simulink model "platform_dp_2021b"  (R2021b)
settings: Solver=ode4  StartTime=0.0  StopTime=500  FixedStep=0.05  RelTol=1e-3
values from neighbouring files (symbols this model uses):
  Kd = 3*alpha_r-beta_r    [kod.m]
  Kd_pos_surge = 0.1    [kod.m]
  Kd_pos_sway = 0.1    [kod.m]
  Ki = alpha_r    [kod.m]
  Ki_vel_surge = alpha_u    [kod.m]
  Ki_vel_sway = alpha_v    [kod.m]
  Kp = 3*alpha_r    [kod.m]
  Kp_pos_surge = 0.05    [kod.m]
  Kp_pos_sway = 0.05    [kod.m]
  Kp_vel_surge = 2*alpha_u    [kod.m]
  Kp_vel_sway = 2*alpha_v    [kod.m]
  limit_max = 2.2    [kod.m]
  limit_min = -limit_max    (= -2.2)    [kod.m]
  pocetni_surge = 1    [kod.m]
  pocetni_sway = 1    [kod.m]
undefined symbols (not defined in the file or in its folder): t200_force, t200_rps
libraries: LABUST_library x7
settings Model: Creator=thor  LastModifiedBy=Filip
settings DataIOCC: SaveFormat=Array  SignalLogging=off  DSMLogging=off  ReturnWorkspaceOutputs=off

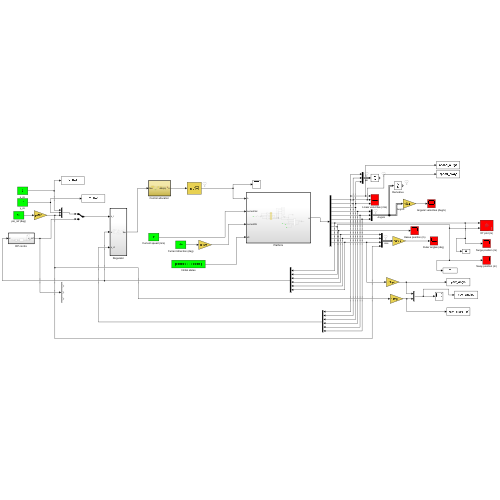
[thumbnail: Simulink's stored preview of the top-level diagram]
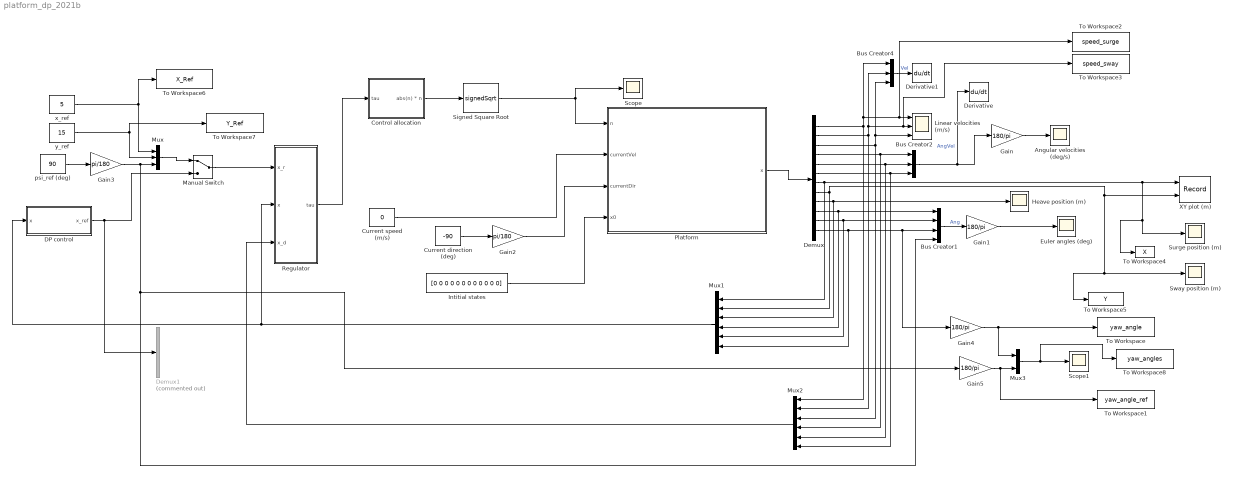
== system platform_dp_2021b ==
  Angular velocities (deg/s) : Scope
  Bus Creator1 : BusCreator  Inputs=4
  Bus Creator2 : BusCreator  Inputs=3
  Bus Creator4 : BusCreator  Inputs=3
  Control allocation : Subsystem  TreatAsAtomicUnit=on
  Current direction (deg) : Constant  Value=-90
  Current speed (m/s) : Constant  Value=0
  DP control : Subsystem  TreatAsAtomicUnit=on
      settings: MinAlgLoopOccurrences=on
  Demux : Demux  Outputs=12
  Demux1 : Demux  Commented=on  Outputs=3
  Derivative : Derivative
  Derivative1 : Derivative
  Euler angles (deg) : Scope
  Gain{,1,4..5} (4 alike) : Gain  Gain=180/pi
  Gain2 : Gain  Gain=pi/180
  Gain3 : Gain  Gain=pi/180
  Heave position (m) : Scope
  Intitial states : Constant  Value=[0 0 0 0 0 0 0 0 0 0 0 0]
  Linear velocities (m/s) : Scope  NumInputPorts=3
  Manual Switch : ManualSwitch
  Mux : Mux  Inputs=3
  Mux1 : Mux  Inputs=6
  Mux2 : Mux  Inputs=6
  Mux3 : Mux  Inputs=2
  Platform : Subsystem  TreatAsAtomicUnit=on
      settings: MinAlgLoopOccurrences=on
  Regulator : Subsystem  TreatAsAtomicUnit=on
  Scope : Scope
  Scope1 : Scope
  Signed Square Root : Sqrt  Operator=signedSqrt  SaturateOnIntegerOverflow=on
  Surge position (m) : Scope
  Sway position (m) : Scope
  To Workspace : ToWorkspace  VariableName=yaw_angle  SaveFormat=Timeseries  SampleTime=-1
  To Workspace1 : ToWorkspace  VariableName=yaw_angle_ref  SaveFormat=Timeseries  SampleTime=-1
  To Workspace2 : ToWorkspace  VariableName=speed_surge  SaveFormat=Timeseries  SampleTime=-1
  To Workspace3 : ToWorkspace  VariableName=speed_sway  SaveFormat=Timeseries  SampleTime=-1
  To Workspace4 : ToWorkspace  VariableName=X  SaveFormat=Timeseries  SampleTime=-1
  To Workspace5 : ToWorkspace  VariableName=Y  SaveFormat=Timeseries  SampleTime=-1
  To Workspace6 : ToWorkspace  VariableName=X_Ref  SaveFormat=Timeseries  SampleTime=-1
  To Workspace7 : ToWorkspace  VariableName=Y_Ref  SaveFormat=Timeseries  SampleTime=-1
  To Workspace8 : ToWorkspace  VariableName=yaw_angles  SaveFormat=Timeseries  SampleTime=-1
  XY plot (m) : Record  FileSettingsInternal="{\"entries\":[{\"content\":{\"excelSettings\":{\"content\":{},\"type\":\"Streamout.ExcelSettings\"}},\"type\":\"Streamout.FileSettingStorage\",\"uuid\":\"f6c939ad-3c6c-47f6-b630-397268ba4e02\"}],\"packageUris\":[\"http://schema.mathworks.com/mf0/streamout_blocks/R2020a\"],\"version\":\"1.0\"}"  Layout=[1 1]  SignalsInternal="{\"entries\":[{\"content\":{\"signals\":[{\"content\":{\"blockPath\":[\"platform_dp_2021b/XY plot (m)\"],\"channel\":[],\"dimensions\":[1],\"domain\":\"platform_dp_2021b/XY plot (m)\",\"lineColor\":\"#a2142f\",\"plots\":[1],\"port\":1,\"sid\":[],\"signalID\":26,\"signalName\":\"Demux:7\"},\"type\":\"RecordBlkView.Signal\",\"uuid\":\"c9e5ced9-c3c6-4cfe-b485-63496ada43a6\"},{\"content\":{\"blockPath\":[\"platform_dp_2021b/XY plot (m)\"],\"channel\":[],\"dimensions\":[1],\"domain\":\"platform_dp_2021b/XY plot (m)\",\"lineColor\":\"#139fff\",\"plots\":[1],\"port\":2,\"sid\":[],\"signalID\":29,\"signalName\":\"Demux:8\"},\"type\":\"RecordBlkView.Signal\",\"uuid\":\"c26e96c1-7e93-4fdd-b2af-f7d2bbcdf98a\"}]},\"type\":\"RecordBlkView.InputSignals\",\"uuid\":\"881e7a22-5157-46d7-a09a-0495ef89bb52\"}],\"packageUris\":[\"http://schema.mathworks.com/mf0/streamout_blocks/R2020a\"],\"version\":\"1.0\"}"  VisualizationBindings="{\"xyplotplugin\":{\"info\":[{\"series\":[{\"bindingParametersList\":[{\"parameter\":\"X-Axis\",\"signalID\":26,\"signalName\":\"Demux:7\"},{\"parameter\":\"Y-Axis\",\"signalID\":29,\"signalName\":\"Demux:8\"}],\"seriesID\":55077}],\"subplotID\":1}]}}"  CompatibilityTag=XY  st=-1
  psi_ref (deg) : Constant  Value=90
  x_ref : Constant  Value=5
  y_ref : Constant  Value=15
  wires:
  Demux/1 -> Bus Creator4/1, To Workspace2/1, Linear velocities (m/s)/1, Mux2/1
  Demux/2 -> To Workspace3/1, Linear velocities (m/s)/2, Bus Creator4/2, Mux2/2
  Demux/3 -> Linear velocities (m/s)/3, Bus Creator4/3, Mux2/3
  Demux/4 -> Mux2/4, Bus Creator2/1
  Demux/5 -> Mux2/5, Bus Creator2/2
  Bus Creator2/1 -> Derivative/1, Gain/1  "AngVel"
  Current speed (m/s)/1 -> Platform/2(currentVel)
  Current direction (deg)/1 -> Gain2/1
  Intitial states/1 -> Platform/4(x0)
  Gain/1 -> Angular velocities (deg/s)/1
  Gain1/1 -> Euler angles (deg)/1
  Gain2/1 -> Platform/3(currentDir)
  Demux/6 -> Mux2/6, Bus Creator2/3
  Gain3/1 -> Mux/3, Gain5/1, Bus Creator1/4
  Bus Creator1/1 -> Gain1/1  "Ang"
  Control allocation/1(abs(n) * n) -> Signed Square Root/1
  Bus Creator4/1 -> Derivative1/1  "Vel"
  y_ref/1 -> To Workspace7/1, Mux/2
  Mux2/1 -> Regulator/3(x_d)
  Platform/1(x) -> Demux/1
  Signed Square Root/1 -> Platform/1(n), Scope/1
  Regulator/1(tau) -> Control allocation/1(tau)
  Mux/1 -> Manual Switch/1
  Manual Switch/1 -> Regulator/1(x_r)
  DP control/1(x_ref) -> Demux1/1, Manual Switch/2
  Mux1/1 -> DP control/1(x), Regulator/2(x)
  Demux/7 -> Mux1/1, Surge position (m)/1, To Workspace4/1, XY plot (m)/1
  Demux/8 -> To Workspace5/1, Sway position (m)/1, XY plot (m)/2, Mux1/2
  Demux/9 -> Mux1/3, Heave position (m)/1
  Demux/10 -> Mux1/4, Bus Creator1/1
  Demux/11 -> Mux1/5, Bus Creator1/2
  Demux/12 -> Mux1/6, Gain4/1, Bus Creator1/3
  psi_ref (deg)/1 -> Gain3/1
  Gain4/1 -> Mux3/1, To Workspace/1
  Mux3/1 -> To Workspace8/1, Scope1/1
  Gain5/1 -> To Workspace1/1, Mux3/2
  x_ref/1 -> To Workspace6/1, Mux/1

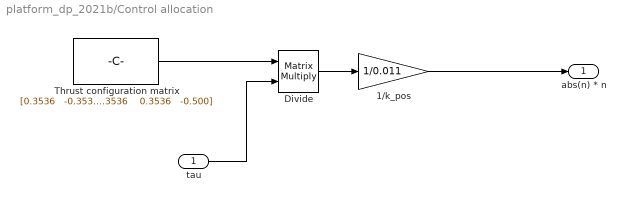
== system platform_dp_2021b/Control allocation ==
  tau : Inport
  1/k_pos : Gain  Gain=1/0.011
  Divide : Product  Inputs=**  Multiplication=Matrix(*)
  Thrust configuration matrix : Constant  Value=|
      | [0.3536   -0.3536   -0.500; 0.3536    0.3536    0.500; -0.3536   -0.3536    0.500
      | ; -0.3536    0.3536   -0.500]
  abs(n) * n : Outport
  wires:
  tau/1 -> Divide/2
  Divide/1 -> 1/k_pos/1
  1/k_pos/1 -> abs(n) * n/1
  Thrust configuration matrix/1 -> Divide/1

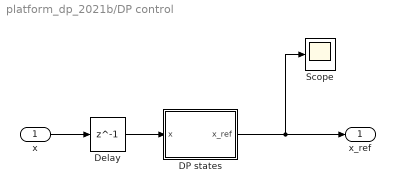
== system platform_dp_2021b/DP control ==
  x : Inport
  DP states : MATLAB Function  TreatAsAtomicUnit=on
  Delay : Delay  DelayLength=1
  Scope : Scope
  x_ref : Outport
  wires:
  x/1 -> Delay/1
  DP states/1(x_ref) -> Scope/1, x_ref/1
  Delay/1 -> DP states/1(x)

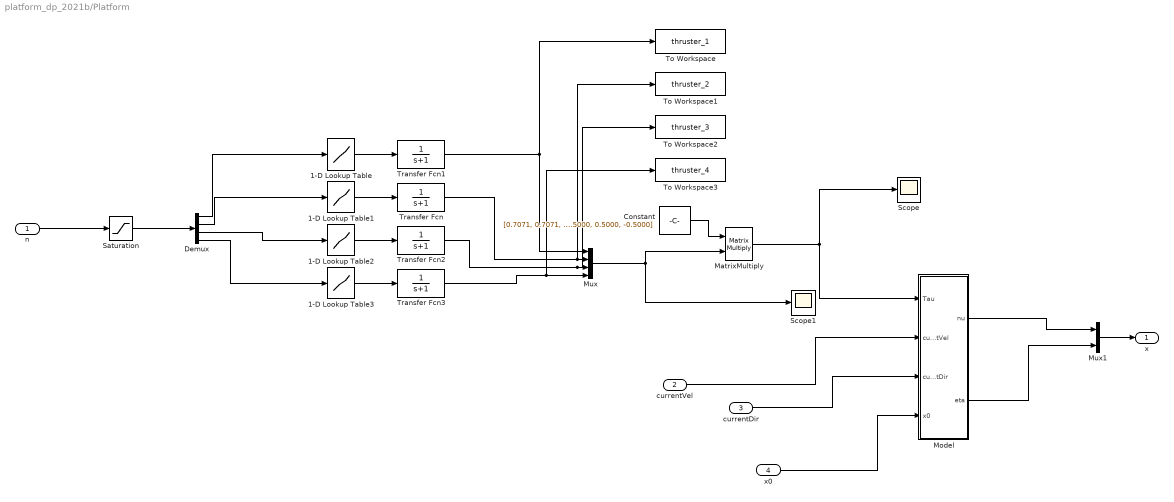
== system platform_dp_2021b/Platform ==
  n : Inport
  currentVel : Inport  Port=2
  currentDir : Inport  Port=3
  x0 : Inport  Port=4
  1-D Lookup Table{,1..3} (4 alike) : Lookup_n-D  NumberOfTableDimensions=1  BreakpointsForDimension1=t200_rps  Table=t200_force  InternalRulePriority=Speed  RndMeth=Simplest  InputSameDT=on
  Constant : Constant  Value="[0.7071, 0.7071, -0.7071, -0.7071; -0.7071,  0.7071, -0.7071,  0.7071; -0.5000, 0.5000, 0.5000, -0.5000]"
  Demux : Demux
  MatrixMultiply : Product  Multiplication=Matrix(*)
  Model : Subsystem
  Mux : Mux
  Mux1 : Mux  Inputs=2
  Saturation : Saturate  UpperLimit=60  LowerLimit=-60
  Scope : Scope
  Scope1 : Scope
  To Workspace : ToWorkspace  VariableName=thruster_1  SaveFormat=Timeseries  SampleTime=-1
  To Workspace1 : ToWorkspace  VariableName=thruster_2  SaveFormat=Timeseries  SampleTime=-1
  To Workspace2 : ToWorkspace  VariableName=thruster_3  SaveFormat=Timeseries  SampleTime=-1
  To Workspace3 : ToWorkspace  VariableName=thruster_4  SaveFormat=Timeseries  SampleTime=-1
  Transfer Fcn{,1..3} (4 alike) : TransferFcn  Denominator=[1 1]
  x : Outport
  wires:
  Transfer Fcn1/1 -> To Workspace/1, Mux/1
  Transfer Fcn/1 -> To Workspace1/1, Mux/2
  Demux/1 -> 1-D Lookup Table/1
  currentVel/1 -> Model/2(currentVel)
  n/1 -> Saturation/1
  Model/1(nu) -> Mux1/1
  Transfer Fcn2/1 -> To Workspace2/1, Mux/3
  Transfer Fcn3/1 -> To Workspace3/1, Mux/4
  Constant/1 -> MatrixMultiply/1
  Mux/1 -> MatrixMultiply/2, Scope1/1
  Model/2(eta) -> Mux1/2
  Mux1/1 -> x/1
  currentDir/1 -> Model/3(currentDir)
  x0/1 -> Model/4(x0)
  MatrixMultiply/1 -> Scope/1, Model/1(Tau)
  Saturation/1 -> Demux/1
  1-D Lookup Table/1 -> Transfer Fcn1/1
  1-D Lookup Table1/1 -> Transfer Fcn/1
  Demux/2 -> 1-D Lookup Table1/1
  Demux/3 -> 1-D Lookup Table2/1
  Demux/4 -> 1-D Lookup Table3/1
  1-D Lookup Table2/1 -> Transfer Fcn2/1
  1-D Lookup Table3/1 -> Transfer Fcn3/1

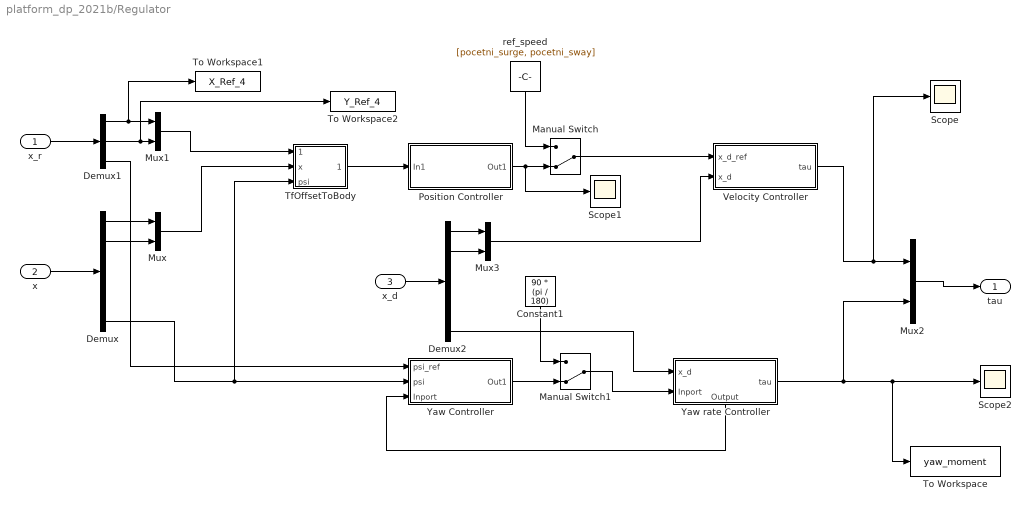
== system platform_dp_2021b/Regulator ==
  x_r : Inport
  x : Inport  Port=2
  x_d : Inport  Port=3
  Constant1 : Constant  Value=90 * (pi / 180)
  Demux : Demux  Outputs=6
  Demux1 : Demux  Outputs=3
  Demux2 : Demux  Outputs=6
  Manual Switch : ManualSwitch  CurrentSetting=0
  Manual Switch1 : ManualSwitch  CurrentSetting=0
  Mux{,1..3} (4 alike) : Mux  Inputs=2
  Position Controller : Subsystem
  Scope : Scope
  Scope1 : Scope
  Scope2 : Scope
  TfOffsetToBody : Subsystem
  To Workspace : ToWorkspace  VariableName=yaw_moment  SaveFormat=Timeseries  SampleTime=-1
  To Workspace1 : ToWorkspace  VariableName=X_Ref_4  SaveFormat=Timeseries  SampleTime=-1
  To Workspace2 : ToWorkspace  VariableName=Y_Ref_4  SaveFormat=Timeseries  SampleTime=-1
  Velocity Controller : Subsystem
  Yaw Controller : Subsystem
  Yaw rate Controller : Subsystem
      settings: PortSchema="{\"entries\":[{\"content\":{\"sides\":[{\"content\":{\"connectorIds\":[\"In1\",\"In2\"]},\"type\":\"ConnectorPlacement.EquallySpacedRectSide\",\"uuid\":\"a08ad913-1b5f-4804-936b-9df89e924933\"},{\"content\":{\"connectorIds\":[\"Out1\"],\"side\":\"RIGHT\"},\"type\":\"ConnectorPlacement.EquallySpacedRectSide\",\"uuid\":\"6b85309d-1e4c-4a26-aaae-a68e51ddcc12\"},{\"content\":{\"connectorIds\":[],\"side\":\"TOP\"},\"type\":\"ConnectorPlacement.EquallySpacedRectSide\",\"uuid\":\"52d97ae7-08e9-4468-b813-b96210971f31\"},{\"content\":{\"connectorIds\":[\"Out2\"],\"side\":\"BOTTOM\"},\"type\":\"ConnectorPlacement.EquallySpacedRectSide\",\"uuid\":\"7dbeefe3-e37d-4eaa-a945-6bd75ab68883\"}]},\"type\":\"ConnectorPlacement.EquallySpacedConnector\",\"uuid\":\"70f5cb1b-651c-4d9e-bb57-ada13c3f9021\"}],\"packageUris\":[\"http://schema.mathworks.com/mf0/Connector/R2020b\"],\"version\":\"1.0\"}"
  ref_speed : Constant  Value=[pocetni_surge, pocetni_sway]
  tau : Outport
  wires:
  TfOffsetToBody/1(Out1) -> Position Controller/1(In1)
  Manual Switch/1 -> Velocity Controller/1(x_d_ref)
  Velocity Controller/1(tau) -> Scope/1, Mux2/1
  Mux3/1 -> Velocity Controller/2(x_d)
  x/1 -> Demux/1
  Demux/1 -> Mux/1
  Demux/2 -> Mux/2
  Mux/1 -> TfOffsetToBody/2(x)
  x_r/1 -> Demux1/1
  Demux1/2 -> To Workspace2/1, Mux1/2
  Mux1/1 -> TfOffsetToBody/1(x_ref)
  Yaw rate Controller/1(tau) -> To Workspace/1, Scope2/1, Mux2/2
  Demux1/3 -> Yaw Controller/1(psi_ref)
  Mux2/1 -> tau/1
  Demux/6 -> TfOffsetToBody/3(psi), Yaw Controller/2(psi)
  Demux2/1 -> Mux3/1
  x_d/1 -> Demux2/1
  Demux2/2 -> Mux3/2
  Demux1/1 -> To Workspace1/1, Mux1/1
  Position Controller/1(Out1) -> Scope1/1, Manual Switch/2
  ref_speed/1 -> Manual Switch/1
  Constant1/1 -> Manual Switch1/1
  Yaw rate Controller/2(Output) -> Yaw Controller/3(Inport)
  Demux2/6 -> Yaw rate Controller/1(x_d)
  Yaw Controller/1(Out1) -> Manual Switch1/2
  Manual Switch1/1 -> Yaw rate Controller/2(Inport)

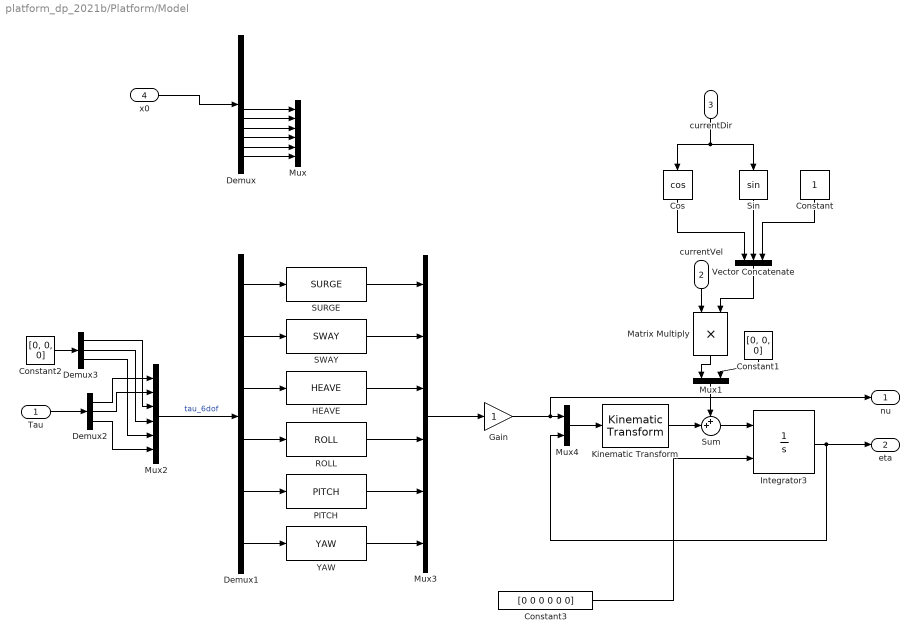
== system platform_dp_2021b/Platform/Model ==
  Tau : Inport
  currentVel : Inport  Port=2
  currentDir : Inport  Port=3
  x0 : Inport  Port=4
  " HEAVE" : LABUST_library/Vehicles/Uncoupled 6DOF/ HEAVE  SystemSampleTime=-1  VariantActivationTime=update diagram  Latency=0  AutoFrameSizeCalculation=off
  " PITCH" : LABUST_library/Vehicles/Uncoupled 6DOF/ PITCH  SystemSampleTime=-1  VariantActivationTime=update diagram  Latency=0  AutoFrameSizeCalculation=off
  " ROLL" : LABUST_library/Vehicles/Uncoupled 6DOF/ ROLL  SystemSampleTime=-1  VariantActivationTime=update diagram  Latency=0  AutoFrameSizeCalculation=off
  " SURGE" : LABUST_library/Vehicles/Uncoupled 6DOF/ SURGE  SystemSampleTime=-1  VariantActivationTime=update diagram  Latency=0  AutoFrameSizeCalculation=off
  " SWAY" : LABUST_library/Vehicles/Uncoupled 6DOF/ SWAY  SystemSampleTime=-1  VariantActivationTime=update diagram  Latency=0  AutoFrameSizeCalculation=off
  " YAW" : LABUST_library/Vehicles/Uncoupled 6DOF/ YAW  SystemSampleTime=-1  VariantActivationTime=update diagram  Latency=0  AutoFrameSizeCalculation=off
  Constant : Constant
  Constant1 : Constant  Value=[0, 0, 0]
  Constant2 : Constant  Value=[0, 0, 0]
  Constant3 : Constant  Value=[0 0 0 0 0 0]
  Cos : Trigonometry  Operator=cos
  Demux : Demux  Outputs=12
  Demux1 : Demux  Outputs=6
  Demux2 : Demux  Outputs=3
  Demux3 : Demux  Outputs=3
  Gain : Gain
  Integrator3 : Integrator  InitialConditionSource=external
  Kinematic Transform : LABUST_library/Vehicles/Uncoupled 6DOF/Kinematic Transform  SystemSampleTime=-1  VariantActivationTime=update diagram  Latency=0  AutoFrameSizeCalculation=off
  Matrix Multiply : Product
  Mux : Mux  Inputs=6
  Mux1 : Mux  Inputs=2
  Mux2 : Mux  Inputs=6
  Mux3 : Mux  Inputs=6
  Mux4 : Mux  Inputs=2
  Sin : Trigonometry
  Sum : Sum  Inputs=++|
  Vector Concatenate : Concatenate  NumInputs=3
  nu : Outport
  eta : Outport  Port=2
  wires:
  Demux1/1 -> " SURGE"/1
  " PITCH"/1 -> Mux3/5
  Mux3/1 -> Gain/1
  " SURGE"/1 -> Mux3/1
  Sum/1 -> Integrator3/1
  Demux1/5 -> " PITCH"/1
  Integrator3/1 -> Mux4/2, eta/1
  Demux1/3 -> " HEAVE"/1
  " HEAVE"/1 -> Mux3/3
  Mux4/1 -> Kinematic Transform/1
  Demux1/4 -> " ROLL"/1
  Demux1/2 -> " SWAY"/1
  " YAW"/1 -> Mux3/6
  Kinematic Transform/1 -> Sum/2
  Gain/1 -> Mux4/1, nu/1
  Demux1/6 -> " YAW"/1
  " SWAY"/1 -> Mux3/2
  " ROLL"/1 -> Mux3/4
  currentVel/1 -> Matrix Multiply/1
  x0/1 -> Demux/1
  currentDir/1 -> Cos/1, Sin/1
  Cos/1 -> Vector Concatenate/1
  Sin/1 -> Vector Concatenate/2
  Constant/1 -> Vector Concatenate/3
  Vector Concatenate/1 -> Matrix Multiply/2
  Demux/7 -> Mux/1
  Demux/8 -> Mux/2
  Demux/9 -> Mux/3
  Demux/10 -> Mux/4
  Demux/11 -> Mux/5
  Demux/12 -> Mux/6
  Matrix Multiply/1 -> Mux1/1
  Constant1/1 -> Mux1/2
  Mux1/1 -> Sum/1
  Tau/1 -> Demux2/1
  Demux2/1 -> Mux2/1
  Demux2/2 -> Mux2/2
  Demux2/3 -> Mux2/6
  Constant2/1 -> Demux3/1
  Demux3/1 -> Mux2/3
  Demux3/2 -> Mux2/4
  Demux3/3 -> Mux2/5
  Mux2/1 -> Demux1/1  "tau_6dof"
  Constant3/1 -> Integrator3/2

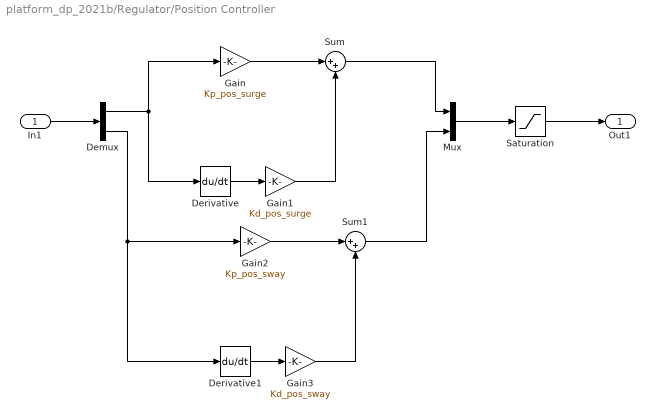
== system platform_dp_2021b/Regulator/Position Controller ==
  In1 : Inport
  Demux : Demux  Outputs=2
  Derivative : Derivative
  Derivative1 : Derivative
  Gain : Gain  Gain=Kp_pos_surge
  Gain1 : Gain  Gain=Kd_pos_surge
  Gain2 : Gain  Gain=Kp_pos_sway
  Gain3 : Gain  Gain=Kd_pos_sway
  Mux : Mux  Inputs=2
  Saturation : Saturate  UpperLimit=2.2  LowerLimit=-2.2
  Sum : Sum  Inputs=|++
  Sum1 : Sum  Inputs=|++
  Out1 : Outport
  wires:
  In1/1 -> Demux/1
  Demux/1 -> Derivative/1, Gain/1
  Derivative/1 -> Gain1/1
  Sum/1 -> Mux/1
  Gain3/1 -> Sum1/2
  Demux/2 -> Derivative1/1, Gain2/1
  Derivative1/1 -> Gain3/1
  Sum1/1 -> Mux/2
  Gain2/1 -> Sum1/1
  Gain/1 -> Sum/1
  Gain1/1 -> Sum/2
  Saturation/1 -> Out1/1
  Mux/1 -> Saturation/1

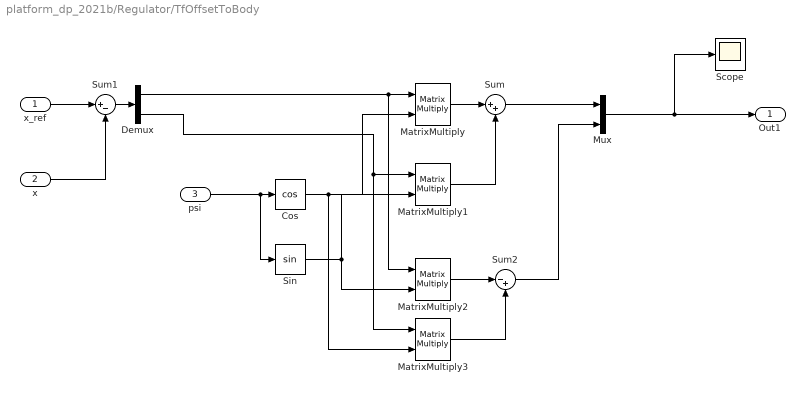
== system platform_dp_2021b/Regulator/TfOffsetToBody ==
  x_ref : Inport
  x : Inport  Port=2
  psi : Inport  Port=3
  Cos : Trigonometry  Operator=cos
  Demux : Demux  Outputs=2
  MatrixMultiply{,1..3} (4 alike) : Product  Multiplication=Matrix(*)
  Mux : Mux  Inputs=2
  Scope : Scope
  Sin : Trigonometry
  Sum : Sum  Inputs=|++
  Sum1 : Sum  Inputs=|+-
  Sum2 : Sum  Inputs=|-+
  Out1 : Outport
  wires:
  psi/1 -> Sin/1, Cos/1
  Cos/1 -> MatrixMultiply/2, MatrixMultiply3/2
  MatrixMultiply/1 -> Sum/1
  Sin/1 -> MatrixMultiply2/2, MatrixMultiply1/2
  MatrixMultiply1/1 -> Sum/2
  Sum/1 -> Mux/1
  Mux/1 -> Scope/1, Out1/1
  x/1 -> Sum1/2
  x_ref/1 -> Sum1/1
  Sum1/1 -> Demux/1
  MatrixMultiply2/1 -> Sum2/1
  MatrixMultiply3/1 -> Sum2/2
  Sum2/1 -> Mux/2
  Demux/1 -> MatrixMultiply2/1, MatrixMultiply/1
  Demux/2 -> MatrixMultiply3/1, MatrixMultiply1/1

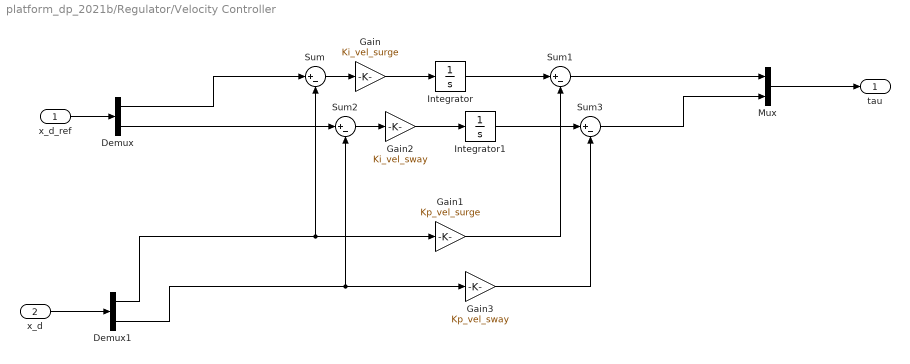
== system platform_dp_2021b/Regulator/Velocity Controller ==
  x_d_ref : Inport
  x_d : Inport  Port=2
  Demux : Demux  Outputs=2
  Demux1 : Demux  Outputs=2
  Gain : Gain  Gain=Ki_vel_surge
  Gain1 : Gain  Gain=Kp_vel_surge
  Gain2 : Gain  Gain=Ki_vel_sway
  Gain3 : Gain  Gain=Kp_vel_sway
  Integrator : Integrator
  Integrator1 : Integrator
  Mux : Mux  Inputs=2
  Sum{,1..3} (4 alike) : Sum  Inputs=|+-
  tau : Outport
  wires:
  x_d/1 -> Demux1/1
  Gain1/1 -> Sum1/2
  Demux1/1 -> Sum/2, Gain1/1
  Sum/1 -> Gain/1
  Gain/1 -> Integrator/1
  Integrator/1 -> Sum1/1
  Sum1/1 -> Mux/1
  Demux/1 -> Sum/1
  Integrator1/1 -> Sum3/1
  Gain3/1 -> Sum3/2
  Demux1/2 -> Sum2/2, Gain3/1
  Demux/2 -> Sum2/1
  Sum3/1 -> Mux/2
  Sum2/1 -> Gain2/1
  Gain2/1 -> Integrator1/1
  Mux/1 -> tau/1
  x_d_ref/1 -> Demux/1

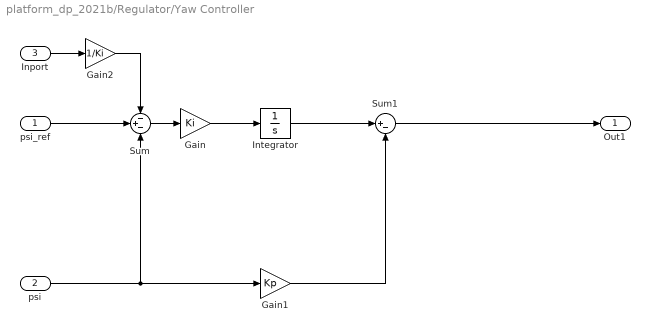
== system platform_dp_2021b/Regulator/Yaw Controller ==
  psi_ref : Inport
  psi : Inport  Port=2
  Inport : Inport  Port=3
  Gain : Gain  Gain=Ki
  Gain1 : Gain  Gain=Kp
  Gain2 : Gain  Gain=1/Ki
  Integrator : Integrator
  Sum : Sum  Inputs=-+-
  Sum1 : Sum  Inputs=|+-
  Out1 : Outport
  wires:
  Sum1/1 -> Out1/1
  Gain/1 -> Integrator/1
  psi/1 -> Gain1/1, Sum/3
  Sum/1 -> Gain/1
  Gain1/1 -> Sum1/2
  Inport/1 -> Gain2/1
  Integrator/1 -> Sum1/1
  psi_ref/1 -> Sum/2
  Gain2/1 -> Sum/1

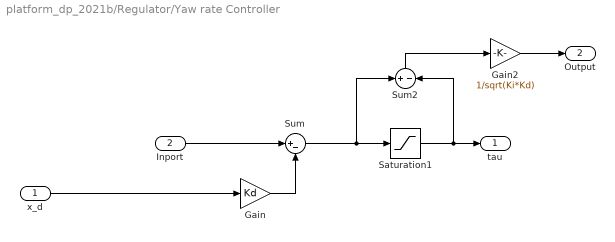
== system platform_dp_2021b/Regulator/Yaw rate Controller ==
  x_d : Inport
  Inport : Inport  Port=2
  Gain : Gain  Gain=Kd
  Gain2 : Gain  Gain=1/sqrt(Ki*Kd)
  Saturation1 : Saturate  UpperLimit=limit_max  LowerLimit=limit_min
  Sum : Sum  Inputs=|+-
  Sum2 : Sum  Inputs=+-
  tau : Outport
  Output : Outport  Port=2
  wires:
  x_d/1 -> Gain/1
  Sum/1 -> Sum2/1, Saturation1/1
  Inport/1 -> Sum/1
  Gain/1 -> Sum/2
  Saturation1/1 -> Sum2/2, tau/1
  Gain2/1 -> Output/1
  Sum2/1 -> Gain2/1

== matlab function platform_dp_2021b/DP control/DP states ==
  data: x input; x_ref output
function x_ref = fcn(x)

references = [
    10 0 0;
    10 10 90;
    0 10 180;
    0 0 360;
];

positionTol = 0.2;
angleTolDeg = 2;


references(:, 3) = references(:, 3) * pi / 180;
angleTol = angleTolDeg * pi / 180;


persistent state;
if isempty(state)
    state = 1;
end

if state > length(references)
    x_ref = [0, 0, 0];
    return
end

currRef = references(state, :);

pos_ref = currRef(1:2);
ang_ref = currRef(3);
pos = x(1:2);
ang = x(6);
if all(abs(pos' - pos_ref) < positionTol, 'all') && abs(ang - ang_ref) < angleTol
    state = state + 1;
    if state > length(references)
        x_ref = [0, 0, 0];
        return
    end
end


x_ref = references(state, :);

end
